simulink model "Blocks_Simlink"  (R2021a)
settings: Solver=VariableStepAuto  StartTime=0.0  StopTime=10.0  RelTol=1e-3
settings Model: Creator=hadee  LastModifiedBy=hadee

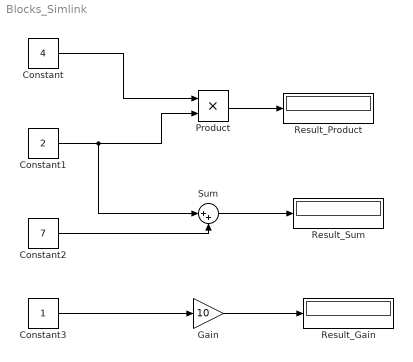
== system Blocks_Simlink ==
  Constant : Constant  Value=4
  Constant1 : Constant  Value=2
  Constant2 : Constant  Value=7
  Constant3 : Constant
  Gain : Gain  Gain=10
  Product : Product
  Result_Gain : Display
  Result_Product : Display
  Result_Sum : Display
  Sum : Sum  Inputs=|++
  wires:
  Constant/1 -> Product/1
  Constant1/1 -> Sum/1, Product/2
  Constant2/1 -> Sum/2
  Constant3/1 -> Gain/1
  Product/1 -> Result_Product/1
  Sum/1 -> Result_Sum/1
  Gain/1 -> Result_Gain/1
